simulink model "Direct_Yaw_Moment_Control_LQR"  (R2018a)
settings: Solver=VariableStepAuto  StartTime=0.0  StopTime=10.0  RelTol=1e-3
model workspace (MATLAB code in the model file):
  | cr=198000;
  | cf=470000;
  | Mz=1000;
  | DeltaF=1;
  | lf=3.67;
  | lr=1.93;
  | m=9950;
  | mu=0.8;
  | v=80;
  | Iz=5;
  | A1=[(-mu*cf-mu*cr)/(m*v) -1+((mu*cr*lr-mu*cf*lf)/(m*v^2))];
  | A2=[(mu*cr*lr-mu*cf*lf)/(Iz) (-mu*cf*lf^2-mu*cr*lr^2)/(Iz*v)];
  | A=[A1;A2];
  | B=[(mu*cf)/(m*v) 0;(mu*cf*lf)/(Iz) 1/Iz];
  | C=[1 0;0 1];
  | D=[0 0;0 0];
  | Q=[1 0;0 10000];
  | R=[0.1 0;0 0.1];
  | K=lqr(A,B,Q,R)
settings Model: Creator=uzeyi  LastModifiedBy=uzeyi

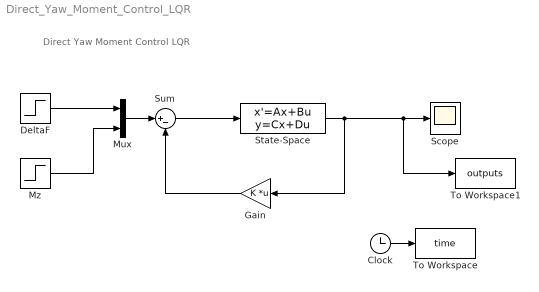
== system Direct_Yaw_Moment_Control_LQR ==
  note: Direct Yaw Moment Control LQR
  Clock : Clock
  DeltaF : Step  After=DeltaF  SampleTime=0
  Gain : Gain  Gain=K  Multiplication=Matrix(K*u)
  Mux : Mux  Inputs=2
  Mz : Step  After=Mz  SampleTime=0
  Scope : Scope
  State-Space : StateSpace  A=A  B=B  C=C  D=[0 0;0 0]  InitialCondition=0
  Sum : Sum  Inputs=|+-
  To Workspace : ToWorkspace  VariableName=time  SampleTime=-1
  To Workspace1 : ToWorkspace  VariableName=outputs  SampleTime=-1
  wires:
  Mux/1 -> Sum/1
  State-Space/1 -> To Workspace1/1, Scope/1, Gain/1
  Sum/1 -> State-Space/1
  DeltaF/1 -> Mux/1
  Gain/1 -> Sum/2
  Mz/1 -> Mux/2
  Clock/1 -> To Workspace/1
